simulink model "raspi_temptest"  (R2020b)
settings: Solver=FixedStepDiscrete  StartTime=0.0  StopTime=inf  RelTol=1e-3
settings Model: ModifiedByFormat=The MathWorks Inc.  Creator=The MathWorks, Inc.  LastModifiedBy=The MathWorks Inc.
settings SolverCC: PositivePriorityOrder=on
settings DataIOCC: LimitDataPoints=on  SaveFormat=Array  ReturnWorkspaceOutputs=off
settings OptimizationCC: LifeSpan=1  MaxStackSize=64
settings DebuggingCC: MergeDetectMultiDrivingBlocksExec=none  SolverPrmCheckMsg=warning  AllowSymbolicDim=off  SFUnexpectedBacktrackingDiag=warning  SFNoUnconditionalDefaultTransitionDiag=warning  SFExecutionAtInitializationDiag=none  ArithmeticOperatorsInVariantConditions=warning
settings HardwareCC: ProdBitPerPointer=32  ProdBitPerSizeT=32  ProdBitPerPtrDiffT=32  ProdLargestAtomicInteger=Long  ProdLargestAtomicFloat=Double  ProdWordSize=32  ProdHWDeviceType=ARM Compatible->ARM Cortex  UseEmbeddedCoderFeatures=off  UseSimulinkCoderFeatures=off
settings ModelReferenceCC: PropagateSignalLabelsOutOfModel=off
settings SFSimCC: SimUseLocalCustomCode=off  MATLABDynamicMemAlloc=off  CustomCodeUndefinedFunction=UseInterfaceOnly
settings RTWCC: Description=Embedded Coder  SystemTargetFile=ert.tlc  HardwareBoard=Raspberry Pi  TemplateMakefile=ert_default_tmf  RTWUseLocalCustomCode=off  Toolchain=GNU GCC Raspberry Pi
settings CodeAppCC: MangleLength=10  StateflowObjectComments=on
settings ERTTargetCC: MultiwordLength=2048  ERTCustomFileBanners=off  SupportContinuousTime=on  SupportNonInlinedSFcns=on  RemoveResetFunc=off  ModelStepFunctionPrototypeControlCompliant=off  ConvertIfToSwitch=off  SuppressUnreachableDefaultCases=off
settings ConfigComp: CovMetricSettings=dw  CovSaveCumulativeToWorkspaceVar=on  CovSaveSingleToWorkspaceVar=on  CovExternalEMLEnable=off  CovSFcnEnable=off

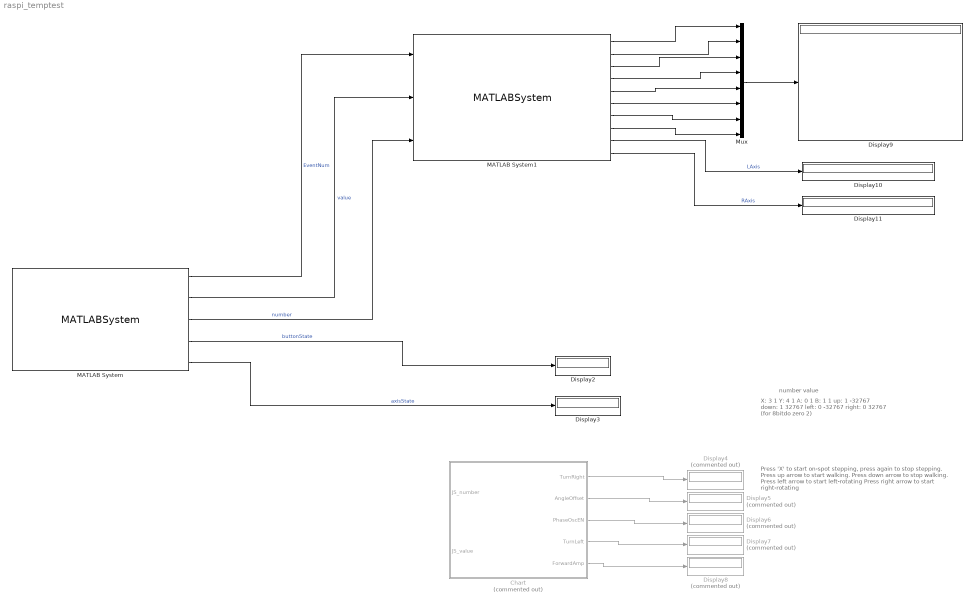
== system raspi_temptest ==
  note: number value
  note: X:            3                                   1
      | Y:            4                                   1
      | A:            0                                   1
      | B:            1                                   1
      | up:           1                               -32767
      | down:      1                                32767
      | left:          0                                -32767
      | right:        0                               32767
      | (for 8bitdo zero 2)
  note: Press 'X' to start on-spot stepping, press again to stop stepping.
      | Press up arrow to start walking.
      | Press down arrow to stop walking.
      | Press left arrow to start left-rotating
      | Press right arrow to start right-rotating
  Chart : Stateflow chart  Commented=on  TreatAsAtomicUnit=on
  Display{2..3,9..11} (5 alike) : Display
      Display2 settings: Format=binary (Stored Integer)
      Display3 settings: Format=binary (Stored Integer)
  Display{4..8} (5 alike) : Display  Commented=on
  MATLAB System : MATLABSystem  System=JoystickRead  SampleTime=0.005
      mask Type: JoystickRead
      mask Display:
      | disp(['Bluetooth' char(10) ' Joystick Reader']);
      | port_label('output',1,'EventNum');
      | port_label('output',2,'value');
      | port_label('output',3,'number');
      | port_label('output',4,'buttonState');
      | port_label('output',5,'axisState');
  MATLAB System1 : MATLABSystem  System=buttonDecoder_2  SimulateUsing=Code generation
      mask Type: buttonDecoder_2
      mask Display:
      | disp('buttonDecoder_2');
      | port_label('input',1,'Eventnum');
      | port_label('input',2,'value');
      | port_label('input',3,'number');
      | port_label('output',1,'X');
      | port_label('output',2,'Y');
      | port_label('output',3,'A');
      | port_label('output',4,'B');
      | port_label('output',5,'up');
      | port_label('output',6,'down');
      | port_label('output',7,'left');
      | port_label('output',8,'right');
      | port_label('output',9,'LAxis');
      | port_label('output',10,'RAxis');
  Mux : Mux  Inputs=8
  wires:
  Chart/1(TurnRight) -> Display4/1
  Chart/2(AngleOffset) -> Display5/1
  Chart/3(PhaseOscEN) -> Display6/1
  Chart/4(TurnLeft) -> Display7/1
  Chart/5(ForwardAmp) -> Display8/1
  MATLAB System1/1 -> Mux/1
  MATLAB System1/2 -> Mux/2
  MATLAB System1/3 -> Mux/3
  MATLAB System1/4 -> Mux/4
  MATLAB System1/5 -> Mux/5
  MATLAB System1/6 -> Mux/6
  MATLAB System1/7 -> Mux/7
  MATLAB System1/8 -> Mux/8
  Mux/1 -> Display9/1
  MATLAB System1/9 -> Display10/1  "LAxis"
  MATLAB System1/10 -> Display11/1  "RAxis"
  MATLAB System/5 -> Display3/1  "axisState"
  MATLAB System/4 -> Display2/1  "buttonState"
  MATLAB System/1 -> MATLAB System1/1  "EventNum"
  MATLAB System/2 -> MATLAB System1/2  "value"
  MATLAB System/3 -> MATLAB System1/3  "number"

== stateflow chart raspi_temptest/Chart ==
  state TurnRight
    entry:
    TurnLeft=0;
    TurnRight=1;
  state Forward
    entry:
    PhaseOscEN=1;
    ForwardAmp=1;
    AngleOffset=0;
    TurnLeft=0;
    TurnRight=0;
  state StandBy
    entry:
    PhaseOscEN=0;
    ForwardAmp=0;
    AngleOffset=0;
    TurnLeft=0;
    TurnRight=0;
  state ClearAngle
    entry:
    AngleOffset=1;
  state OnSpot
    entry:
    PhaseOscEN=1;
    ForwardAmp=0;
    AngleOffset=0;
    TurnLeft=0;
    TurnRight=0;
  state TurnLeft
    entry:
    TurnLeft=1;
    TurnRight=0;
  OnSpot -> TurnRight [order 2] : [JS_number==0 && JS_value>1000]
  TurnRight -> OnSpot [order 2] : [JS_number==0 && JS_value<-1000 && ForwardAmp==0]
  Forward -> TurnRight [order 1] : [JS_number==0 && JS_value>1000]
  TurnRight -> Forward [order 1] : [JS_number==0 && JS_value<-1000 && ForwardAmp==1]
  (default) -> StandBy
  OnSpot -> Forward [order 1] : [JS_number==1 && JS_value<-1000]
  ClearAngle -> OnSpot : after(1,sec)
  StandBy -> ClearAngle : [JS_number==3 && JS_value==1]
  TurnLeft -> Forward [order 1] : [JS_number==0 && JS_value>1000 && ForwardAmp==1]
  Forward -> OnSpot [order 3] : [JS_number==1 && JS_value>1000]
  Forward -> TurnLeft [order 2] : [JS_number==0 && JS_value<-1000]
  OnSpot -> StandBy [order 3] : [JS_number==3 && JS_value==1]
  OnSpot -> TurnLeft [order 4] : [JS_number==0 && JS_value<-1000]
  TurnLeft -> OnSpot [order 2] : [JS_number==0 && JS_value>1000 && ForwardAmp==0]
  data: JS_number input; JS_value input; TurnRight output; AngleOffset output; PhaseOscEN output; TurnLeft output; ForwardAmp output
